simulink model "UAM_Flight_control"  (R2024b)
settings: Solver=FixedStepAuto  StartTime=0.0  StopTime=inf  RelTol=1e-3  EnableMultiTasking=on
undefined symbols (not defined in the file): CityMission, control, controlParams, ControlSampleTime, Cruise_a, DiscIntNeverNeededParam, Earth, FixedWingMission, flightState, FSState, FWControlParams, FWTrimSpeed, HoverMission, params, position, R_WAYPOINTTRANSITION, TransitionMission, uavParam, Vt, w_trim, WGS84, zGround
libraries: slpidlib x56, simulink x35, uavalgslib x8, robotcorelib x2, simulink_extras x2, mspfiltlib x1, aerolibtransform2 x1
(part 2 of 12)

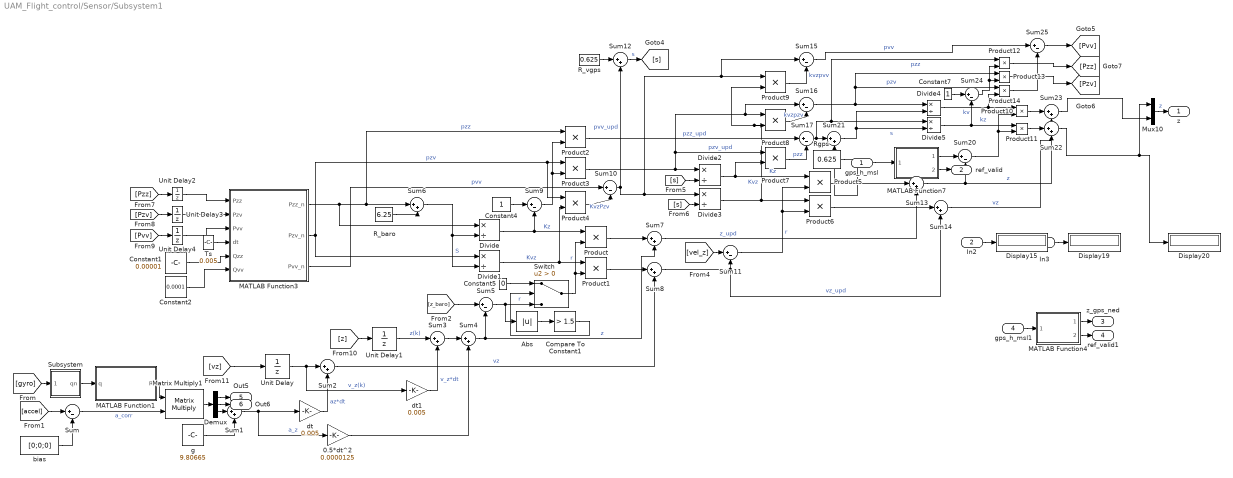
== system UAM_Flight_control/Sensor/Subsystem1 ==
  gps_h_msl : Inport
  In2 : Inport  Port=2
  In3 : Inport  Port=3
  gps_h_msl1 : Inport  Port=4
  0.5*dt^2 : Gain  Gain=0.0000125
  Abs : Abs  SaturateOnIntegerOverflow=off
  Compare To Constant1 : simulink/Logic and Bit Operations/Compare To Constant  relop=>  const=1.5  OutDataTypeStr=boolean
  Constant1 : Constant  Value=0.00001
  Constant2 : Constant  Value=0.0001
  Constant4 : Constant
  Constant5 : Constant  Value=0
  Constant7 : Constant
  Demux : Demux  Outputs=3
  Display15 : Display
  Display19 : Display
  Display20 : Display
  Divide{,1..5} (6 alike) : Product  Inputs=*/
  MATLAB Function1 : MATLAB Function  TreatAsAtomicUnit=on
  MATLAB Function3 : MATLAB Function  TreatAsAtomicUnit=on
  MATLAB Function4 : MATLAB Function  TreatAsAtomicUnit=on
  MATLAB Function7 : MATLAB Function  TreatAsAtomicUnit=on
  Matrix Multiply1 : Product  Multiplication=Matrix(*)
  Mux10 : Mux  Inputs=2
  Product{,1..14} (15 alike) : Product
  R_baro : Constant  Value=6.25
  R_vgps : Constant  Value=0.625
  Rgps : Constant  Value=0.625
  Subsystem : Subsystem
  Sum{,5,9..11,15..17,20,24..25} (11 alike) : Sum  Inputs=|+-
  Sum{1..4,6..8,12..14,21..23} (13 alike) : Sum  Inputs=|++
  Switch : Switch  Criteria=u2 > Threshold  SaturateOnIntegerOverflow=off  InputSameDT=off
  Ts : Constant  Value=0.005
  Unit Delay{,1..4} (5 alike) : UnitDelay  SampleTime=-1  HasFrameUpgradeWarning=on
  bias : Constant  Value=[0;0;0]
  dt : Gain  Gain=0.005
  dt1 : Gain  Gain=0.005
  g : Constant  Value=9.80665
  z : Outport
  ref_valid : Outport  Port=2
  z_gps_ned : Outport  Port=3
  ref_valid1 : Outport  Port=4
  Out5 : Outport  Port=5
  Out6 : Outport  Port=6
  wires:
  Sum1/1 -> dt/1, 0.5*dt^2/1  "a_z"
  Sum10/1 -> Sum12/2, Product9/1, Sum15/1, Divide3/1  "pvv_upd"
  In2/1 -> Display15/1
  Constant5/1 -> Switch/1
  Sum6/1 -> Divide1/2, Divide/2  "S"
  Unit Delay/1 -> dt1/1, Sum2/1  "v_z(k)"
  gps_h_msl1/1 -> MATLAB Function4/1(gps_h_msl)
  Divide2/1 -> Product7/2, Product5/1  "Kz"
  Product9/1 -> Sum15/2  "kvzpvv"
  Sum16/1 -> Product13/1, Product14/1, Divide4/1  "pzv"
  dt1/1 -> Sum3/2  "v_z*dt"
  [vz] -> Unit Delay/1
  [Pzv] -> Unit Delay3/1
  Divide4/1 -> Product14/2, Product10/1  "kv"
  Ts/1 -> MATLAB Function3/4(dt)
  bias/1 -> Sum/2
  Sum13/1 -> Sum22/2, Sum20/2  "z"
  MATLAB Function7/1(z_gps_ned) -> Sum20/1
  Matrix Multiply1/1 -> Demux/1
  [Pzz] -> Unit Delay2/1
  Compare To Constant1/1 -> Switch/2
  [z] -> Unit Delay1/1
  g/1 -> Sum1/2
  Sum20/1 -> Product11/2, Product10/2
  Product12/1 -> [Pzz]
  Abs/1 -> Compare To Constant1/1
  Unit Delay2/1 -> MATLAB Function3/1(Pzz)
  Divide3/1 -> Product9/2, Product8/2, Product6/1  "Kvz"
  Sum9/1 -> Product2/2, Product3/2
  Sum/1 -> Matrix Multiply1/2  "a_corr"
  Sum7/1 -> Sum13/2  "z_upd"
  Sum23/1 -> Mux10/2
  Product5/1 -> Sum13/1
  Sum4/1 -> Sum7/2, Sum5/2  "z"
  Sum22/1 -> Display20/1, Mux10/1
  Sum21/1 -> Divide5/2, Divide4/2  "s"
  Sum2/1 -> Sum8/2  "vz"
  R_baro/1 -> Sum6/2
  Sum17/1 -> Product12/1, Divide5/1, Sum21/1  "pzz"
  MATLAB Function3/3(Pvv_n) -> Sum10/1  "pvv"
  dt/1 -> Sum2/2  "az*dt"
  Divide1/1 -> Product1/1, Product4/2  "Kvz"
  Product13/1 -> [Pzv]
  Constant2/1 -> MATLAB Function3/6(Qvv)
  Sum5/1 -> Switch/3, Abs/1  "r"
  Sum25/1 -> [Pvv]
  Product/1 -> Sum7/1
  Sum11/1 -> Product6/2, Product5/2  "r"
  Product10/1 -> Sum23/1
  Sum3/1 -> Sum4/1
  MATLAB Function3/2(Pzv_n) -> Divide1/1, Product4/1, Product3/1  "pzv"
  Sum8/1 -> Sum14/2, Sum11/2  "vz_upd"
  [gyro] -> Subsystem/1(Inport)
  Subsystem/1(qn) -> MATLAB Function1/1(q)
  MATLAB Function7/2(ref_valid) -> ref_valid/1
  [accel] -> Sum/1
  MATLAB Function3/1(Pzz_n) -> Divide/1, Product2/1, Sum6/1  "pzz"
  Product8/1 -> Sum16/2  "kvzpzv"
  Sum15/1 -> Sum25/1  "pvv"
  Product7/1 -> Sum17/2  "pzz"
  Unit Delay4/1 -> MATLAB Function3/3(Pvv)
  Rgps/1 -> Sum21/2
  Divide5/1 -> Product11/1, Sum24/2  "kz"
  Product3/1 -> Sum16/1, Product8/1, Product7/1, Divide2/1  "pzv_upd"
  Switch/1 -> Product/2, Product1/2  "r"
  Product4/1 -> Sum10/2  "KvzPzv"
  Unit Delay3/1 -> MATLAB Function3/2(Pzv)
  Unit Delay1/1 -> Sum3/1  "z(k)"
  Divide/1 -> Sum9/2, Product/1  "Kz"
  [vel_z] -> Sum11/1
  [s] -> Divide2/2
  Product11/1 -> Sum22/1
  Demux/3 -> Sum1/1
  Constant1/1 -> MATLAB Function3/5(Qzz)
  Sum24/1 -> Product13/2, Product12/2
  Constant4/1 -> Sum9/1
  R_vgps/1 -> Sum12/1
  [s] -> Divide3/2
  Sum12/1 -> [s]  "s"
  Product1/1 -> Sum8/1
  Product14/1 -> Sum25/2
  Sum14/1 -> Sum23/2  "vz"
  [Pvv] -> Unit Delay4/1
  Product6/1 -> Sum14/1
  MATLAB Function1/1(R) -> Matrix Multiply1/1
  Product2/1 -> Sum17/1  "pzz_upd"
  0.5*dt^2/1 -> Sum4/2
  Constant7/1 -> Sum24/1
  [z_baro] -> Sum5/1
  gps_h_msl/1 -> MATLAB Function7/1(gps_h_msl)
  In3/1 -> Display19/1
  MATLAB Function4/1(z_gps_ned) -> z_gps_ned/1
  MATLAB Function4/2(ref_valid) -> ref_valid1/1
  Demux/2 -> Out6/1
  Mux10/1 -> z/1  "z"
  Demux/1 -> Out5/1

== system UAM_Flight_control/Sensor/Subsystem2 ==
  fcc : Inport
  In2 : Inport  Port=2
  Constant1 : Constant  Value=0
  Gain : Gain  Gain=pi/180
  Gain1 : Gain  Gain=pi/180
  Matrix Concatenate : Concatenate  NumInputs=3  Mode=Multidimensional array  ConcatenateDimension=2
  Product{,1..3} (4 alike) : Product
  Trigonometric Function : Trigonometry
  Trigonometric Function1 : Trigonometry  Operator=cos
  Trigonometric Function2 : Trigonometry  Operator=cos
  Trigonometric Function3 : Trigonometry
  Unary Minus{,1..5} (6 alike) : UnaryMinus
  Vector Concatenate : Concatenate  NumInputs=3
  Vector Concatenate1 : Concatenate  NumInputs=3
  Vector Concatenate2 : Concatenate  NumInputs=3
  Out1 : Outport
  wires:
  Product3/1 -> Unary Minus3/1
  Vector Concatenate/1 -> Matrix Concatenate/1
  Trigonometric Function1/1 -> Vector Concatenate1/2, Product3/2, Product/2, Product2/2
  Unary Minus4/1 -> Vector Concatenate2/3
  Vector Concatenate2/1 -> Matrix Concatenate/3
  Trigonometric Function3/1 -> Unary Minus5/1, Product1/2
  Trigonometric Function/1 -> Product1/1, Unary Minus4/1, Product/1
  Gain/1 -> Trigonometric Function2/1, Trigonometric Function/1
  Product/1 -> Unary Minus/1
  Vector Concatenate1/1 -> Matrix Concatenate/2
  Trigonometric Function2/1 -> Product2/1, Product3/1, Vector Concatenate/3
  fcc/1 -> Gain/1
  Gain1/1 -> Trigonometric Function1/1, Trigonometric Function3/1
  Constant1/1 -> Vector Concatenate1/3
  Unary Minus5/1 -> Vector Concatenate1/1
  In2/1 -> Gain1/1
  Unary Minus2/1 -> Vector Concatenate2/1
  Product2/1 -> Unary Minus2/1
  Product1/1 -> Unary Minus1/1
  Unary Minus/1 -> Vector Concatenate/1
  Unary Minus1/1 -> Vector Concatenate/2
  Unary Minus3/1 -> Vector Concatenate2/2
  Matrix Concatenate/1 -> Out1/1

== system UAM_Flight_control/Controller/Auto1/Blend Scheduler ==
  note: Forward Transition Tilt Mode Manager
  FlightMode : Inport
  States : Inport  Port=2
  MixerCommands : Inport  Port=3
  BTalpha : Subsystem  TreatAsAtomicUnit=on
  Bus Creator : BusCreator  Inputs=5
  Bus Selector1 : BusSelector  OutputSignals=w_phi,w_theta,w_psi,w_z
  Constant : Constant  Value=flightState.Transition
  Constant2 : Constant  Value=0.25*uavParam.geom.mass*9.81
  Constant3 : Constant  Value=FWTrimSpeed
  Constant4 : Constant  Value=FWTrimSpeed
  Constant5 : Constant
  Constant6 : Constant  Value=78.54
  Constant7 : Constant
  Demux : Demux
  FTalpha : Subsystem
  Gain3 : Gain  Gain=0
  Mux : Mux
  Product1 : Product
  Product2 : Product
  Product3 : Product
  Relational Operator : RelationalOperator  Operator===  OutDataTypeStr=boolean  RndMeth=Simplest  InputSameDT=off
  Subtract : Sum  Inputs=+-
  Subtract1 : Sum  Inputs=+-
  Sum1 : Sum  Inputs=|++
  Sum3 : Sum  Inputs=|+-
  Switch : Switch  Criteria=u2 > Threshold  SaturateOnIntegerOverflow=off  InputSameDT=off
  Switch1 : Switch  Criteria=u2 > Threshold  SaturateOnIntegerOverflow=off  InputSameDT=off
  MotorCommands : Outport
  alpha : Outport  Port=2
  FlightState : Outport  Port=3
  wires:
  FlightMode/1 -> Relational Operator/1, FlightState/1
  Relational Operator/1 -> [trigger]
  Bus Selector1/4 -> Sum1/1  "<w_z>"
  Constant2/1 -> Sum1/2
  [liftblending] -> Product2/2
  Mux/1 -> Product2/1
  MixerCommands/1 -> Bus Selector1/1
  Bus Selector1/1 -> Mux/1  "<w_phi>"
  Bus Selector1/2 -> Mux/2  "<w_theta>"
  Bus Selector1/3 -> Mux/3  "<w_psi>"
  Sum1/1 -> Mux/4  "w_z"
  Product2/1 -> Demux/1
  Demux/1 -> Bus Creator/1  "w_phi"
  Demux/2 -> Bus Creator/2  "w_theta"
  Demux/3 -> Bus Creator/3  "w_psi"
  Demux/4 -> Bus Creator/4  "w_z"
  Bus Creator/1 -> MotorCommands/1
  Constant6/1 -> Product1/1
  States/1 -> FTalpha/1(States), BTalpha/1(States)
  Switch/1 -> [liftblending], Subtract1/2
  FTalpha/1(alpha) -> Switch/1
  BTalpha/1(alpha) -> Switch/3
  [trigger] -> Switch/2
  Product1/1 -> Sum3/2
  Sum3/1 -> Switch1/1  "cruise"
  [trigger] -> Switch1/2
  Switch1/1 -> Bus Creator/5  "cruise"
  Constant3/1 -> Gain3/1
  Gain3/1 -> Product3/1
  Constant5/1 -> Subtract/1
  [liftblending] -> Subtract/2
  Subtract/1 -> Product3/2
  Product3/1 -> Switch1/3
  Constant7/1 -> Subtract1/1
  Subtract1/1 -> alpha/1
  Constant/1 -> Relational Operator/2
  [liftblending] -> Product1/2
  Constant4/1 -> Sum3/1

== system UAM_Flight_control/Controller/Auto1/Fixed Wing Controller ==
  States : Inport
  Control Mode : Inport  Port=2
  AAC SP : Inport  Port=3  OutDataTypeStr=Bus: AAC
  FixedWingSP : Inport  Port=4  OutDataTypeStr=Bus: FixedWingCommandBus
  AERT : Inport  Port=5
  In1 : Inport  Port=6
  Actuator Armed : EnablePort
  Subsystem : Subsystem
  Actuator : Outport
  wires:
  States/1 -> Subsystem/1(States)
  Control Mode/1 -> Subsystem/2(Control Mode)
  AAC SP/1 -> Subsystem/3(AAC SP)
  Subsystem/1(Actuator) -> Actuator/1
  AERT/1 -> Subsystem/5(AERT)
  FixedWingSP/1 -> Subsystem/4(FixedWingSP)
  In1/1 -> Subsystem/6(Intransition)

== system UAM_Flight_control/Controller/Auto1/Manual Control ==
  Bus Creator : BusCreator  Inputs=4
  Constant{,1..3} (4 alike) : Constant  Value=0  SampleTime=-1
  AERT : Outport
  wires:
  Constant/1 -> Bus Creator/1  "aileron"
  Constant1/1 -> Bus Creator/2  "throttle"
  Constant2/1 -> Bus Creator/3  "elevator"
  Constant3/1 -> Bus Creator/4  "rudder"
  Bus Creator/1 -> AERT/1

== system UAM_Flight_control/Controller/Auto1/Multicopter Controller ==
  note: Prefilter
  Hover Commands : Inport  OutDataTypeStr=Bus: HoverSPBus
  States : Inport  Port=2
  InTransition : Inport  Port=3
  CtrlMode : Inport  Port=4
  FlightMode : Inport  Port=5
  " Armed" : EnablePort
  Attitude & Altitude controller : Subsystem
  Demux1 : Demux
  Horizontal Position Control : Subsystem  TreatAsAtomicUnit=on
  Merge : Merge
  Merge1 : Merge
  Mux : Mux  Inputs=3
  NOT1 : Logic  Operator=NOT  IconShape=distinctive  AllPortsSameDT=off  OutDataTypeStr=boolean
  Organize Inputs : Subsystem
  transition controller : Subsystem
  MixerCommands : Outport
  wires:
  Organize Inputs/1(MixerCommands) -> MixerCommands/1
  Demux1/1 -> [XRef]
  [State] -> Horizontal Position Control/3(States)
  Demux1/3 -> [ZRef]
  NOT1/1 -> Horizontal Position Control/Enable
  [XRef] -> Horizontal Position Control/1(XRef)
  [YRef] -> Horizontal Position Control/2(YRef)
  InTransition/1 -> [Transition]
  States/1 -> [State]
  Hover Commands/1 -> Demux1/1
  Demux1/4 -> [YawRef]
  Mux/1 -> Attitude & Altitude controller/1(Ref Attitude)
  [State] -> Attitude & Altitude controller/2(States)
  [ZRef] -> Attitude & Altitude controller/3(Z ref)
  [Transition] -> Attitude & Altitude controller/4(InTransition)
  Attitude & Altitude controller/1(Roll torque cmd) -> Organize Inputs/2(commanded phi torque)
  Attitude & Altitude controller/2(Pitch torque Cmd) -> Organize Inputs/3(commanded theta torque)
  Attitude & Altitude controller/4(commanded thrust) -> Organize Inputs/5(commanded thrust)
  FlightMode/1 -> Attitude & Altitude controller/6(FlightMode)
  Attitude & Altitude controller/3(Yaw torque Cmd) -> Organize Inputs/4(commanded psi torque)
  [Transition] -> NOT1/1, transition controller/Enable
  [YawRef] -> Mux/3
  Demux1/2 -> [YRef]
  Merge/1 -> Mux/1
  Merge1/1 -> Mux/2
  transition controller/1(Rollcmd) -> Merge/2
  transition controller/2(Pitchcmd) -> Merge1/2
  Horizontal Position Control/1(Roll Cmd) -> Merge/1
  Horizontal Position Control/2(Pitch Cmd) -> Merge1/1
  CtrlMode/1 -> Attitude & Altitude controller/5(CtrlMode)

== system UAM_Flight_control/Controller/Auto1/Scheduler ==
  MotorCommands : Inport
  FlightState : Inport  Port=2  OutDataTypeStr=Enum: flightState
  CtrlMode : Inport  Port=3
  FixedWingActuators : Inport  Port=4
  " Armed" : EnablePort
  FixedWingScheduler : Subsystem
  Subsystem : Subsystem
  MotorActuatorCommands : Outport  OutputWhenDisabled=reset  InitialOutput=0
  CtrlSurfaceCommands : Outport  Port=2  OutDataTypeStr=Bus: FixedWingCtrlBus  OutputWhenDisabled=reset  InitialOutput=0  VectorParamsAs1DForOutWhenUnconnected=off
  wires:
  FixedWingScheduler/1(ActuatorControls) -> CtrlSurfaceCommands/1, Subsystem/2(FixedWingActuators)
  FlightState/1 -> Subsystem/1(FlightState), FixedWingScheduler/1(FlightState)
  Subsystem/1(ActuatorControls) -> MotorActuatorCommands/1
  MotorCommands/1 -> Subsystem/4(MotorCommands)
  FixedWingActuators/1 -> FixedWingScheduler/2(FixedWingActuators)
  CtrlMode/1 -> Subsystem/3(CtrlMode)

== system UAM_Flight_control/Controller/Emergency/Blend Scheduler ==
  FlightMode : Inport
  States : Inport  Port=2
  Constant : Constant  Value=flightState.Transition
  Constant1 : Constant  Value=flightState.BackTransition
  Discrete-Time Integrator : DiscreteIntegrator  gainval=0.01  SampleTime=-1  ICPrevOutput=DiscIntNeverNeededParam  ICPrevScaledInput=DiscIntNeverNeededParam
  Gain : Gain
  Gain1 : Gain  Gain=-1
  Relational Operator : RelationalOperator  Operator===  OutDataTypeStr=boolean  RndMeth=Simplest  InputSameDT=off
  Relational Operator1 : RelationalOperator  Operator===  OutDataTypeStr=boolean  RndMeth=Simplest  InputSameDT=off
  Saturation : Saturate  UpperLimit=1  LowerLimit=0  OutDataTypeStr=double
  Sum : Sum  Inputs=|++
  Terminator : Terminator
  alpha : Outport
  FlightState : Outport  Port=2
  wires:
  FlightMode/1 -> Relational Operator1/1, Relational Operator/1, FlightState/1
  Gain/1 -> Sum/1
  Gain1/1 -> Sum/2
  Sum/1 -> Discrete-Time Integrator/1
  Discrete-Time Integrator/1 -> Saturation/1
  Saturation/1 -> alpha/1  "a"
  States/1 -> Terminator/1
  Constant/1 -> Relational Operator/2
  Relational Operator/1 -> Gain/1
  Constant1/1 -> Relational Operator1/2
  Relational Operator1/1 -> Gain1/1

== system UAM_Flight_control/Controller/Emergency/FixedWing Controller ==
  States : Inport
  Control Mode : Inport  Port=2
  RC : Inport  Port=3
  Actuator Armed : EnablePort
  Subsystem : Subsystem
  Actuator : Outport
  wires:
  States/1 -> Subsystem/1(States)
  Control Mode/1 -> Subsystem/2(Control Mode)
  Subsystem/1(Actuator) -> Actuator/1
  RC/1 -> Subsystem/3(RC)

== system UAM_Flight_control/Controller/Emergency/Scheduler ==
  MotorCommands : Inport
  BlendingSchedule : Inport  Port=2
  FlightState : Inport  Port=3  OutDataTypeStr=Enum: flightState
  TransitionDone : Inport  Port=4
  BackTransitionDone : Inport  Port=5
  FixedWingActuators : Inport  Port=6  OutDataTypeStr=Bus: FixedWingCtrlBus
  Actuator Armed : EnablePort
  FixedWingScheduler : Subsystem
  Subsystem : Subsystem
  MotorActuatorCommands : Outport  OutputWhenDisabled=reset  InitialOutput=0
  CtrlSurfaceCommands : Outport  Port=2  OutDataTypeStr=Bus: FixedWingCtrlBus  OutputWhenDisabled=reset  InitialOutput=0  VectorParamsAs1DForOutWhenUnconnected=off
  wires:
  FixedWingScheduler/1(ActuatorControls) -> CtrlSurfaceCommands/1, Subsystem/2(FixedWingActuators)
  FlightState/1 -> Subsystem/1(FlightState), FixedWingScheduler/1(FlightState)
  BlendingSchedule/1 -> Subsystem/4(BlendingSchedule)
  Subsystem/1(ActuatorControls) -> MotorActuatorCommands/1
  MotorCommands/1 -> Subsystem/3(MotorCommands)
  FixedWingActuators/1 -> FixedWingScheduler/2(FixedWingActuators)
  TransitionDone/1 -> Subsystem/5(TransitionDone), FixedWingScheduler/3(TransitionDone)
  BackTransitionDone/1 -> Subsystem/6(BackTransitionDone)

== system UAM_Flight_control/Controller/Emergency/multicopter Controller ==
  RC : Inport
  States : Inport  Port=2
  Actuator Armed : EnablePort
  Attitude & Altitude controller : Subsystem
  Demux : Demux  Outputs=10
  Mux1 : Mux  Inputs=3
  Organize Inputs : Subsystem
  Terminator{,1..6} (7 alike) : Terminator
  MixerCommands : Outport
  wires:
  Demux/6 -> Terminator2/1
  Organize Inputs/1(MixerCommands) -> MixerCommands/1
  Demux/2 -> Organize Inputs/1(forward command), Mux1/2
  Demux/5 -> Terminator1/1
  Attitude & Altitude controller/3(Yaw torque Cmd) -> Organize Inputs/4(commanded psi torque)
  States/1 -> Attitude & Altitude controller/2(States)
  Demux/4 -> Mux1/3
  Attitude & Altitude controller/1(Roll torque cmd) -> Organize Inputs/2(commanded phi torque)
  Attitude & Altitude controller/2(Pitch torque Cmd) -> Organize Inputs/3(commanded theta torque)
  Attitude & Altitude controller/4(commanded thrust) -> Organize Inputs/5(commanded thrust)
  Demux/1 -> Mux1/1
  Mux1/1 -> Attitude & Altitude controller/1(Ref Attitude)
  Demux/3 -> Terminator/1
  RC/1 -> Demux/1
  Demux/7 -> Terminator3/1
  Demux/8 -> Terminator4/1
  Demux/9 -> Terminator5/1
  Demux/10 -> Terminator6/1

== system UAM_Flight_control/Controller/Manual/Blend Scheduler ==
  FlightMode : Inport
  States : Inport  Port=2
  Constant : Constant  Value=flightState.Transition
  Constant1 : Constant  Value=flightState.BackTransition
  Discrete-Time Integrator : DiscreteIntegrator  gainval=0.01  SampleTime=-1  ICPrevOutput=DiscIntNeverNeededParam  ICPrevScaledInput=DiscIntNeverNeededParam
  Gain : Gain
  Gain1 : Gain  Gain=-1
  Relational Operator : RelationalOperator  Operator===  OutDataTypeStr=boolean  RndMeth=Simplest  InputSameDT=off
  Relational Operator1 : RelationalOperator  Operator===  OutDataTypeStr=boolean  RndMeth=Simplest  InputSameDT=off
  Saturation : Saturate  UpperLimit=1  LowerLimit=0  OutDataTypeStr=double
  Sum : Sum  Inputs=|++
  Terminator : Terminator
  alpha : Outport
  FlightState : Outport  Port=2
  wires:
  FlightMode/1 -> Relational Operator1/1, Relational Operator/1, FlightState/1
  Gain/1 -> Sum/1
  Gain1/1 -> Sum/2
  Sum/1 -> Discrete-Time Integrator/1
  Discrete-Time Integrator/1 -> Saturation/1
  Saturation/1 -> alpha/1  "a"
  States/1 -> Terminator/1
  Constant/1 -> Relational Operator/2
  Relational Operator/1 -> Gain/1
  Constant1/1 -> Relational Operator1/2
  Relational Operator1/1 -> Gain1/1

== system UAM_Flight_control/Controller/Manual/FixedWing Controller ==
  States : Inport
  Control Mode : Inport  Port=2
  RC : Inport  Port=3
  Actuator Armed : EnablePort
  Subsystem : Subsystem
  Actuator : Outport
  wires:
  States/1 -> Subsystem/1(States)
  Control Mode/1 -> Subsystem/2(Control Mode)
  Subsystem/1(Actuator) -> Actuator/1
  RC/1 -> Subsystem/3(RC)

== system UAM_Flight_control/Controller/Manual/Scheduler ==
  MotorCommands : Inport
  BlendingSchedule : Inport  Port=2
  FlightState : Inport  Port=3  OutDataTypeStr=Enum: flightState
  TransitionDone : Inport  Port=4
  BackTransitionDone : Inport  Port=5
  FixedWingActuators : Inport  Port=6  OutDataTypeStr=Bus: FixedWingCtrlBus
  Actuator Armed : EnablePort
  FixedWingScheduler : Subsystem
  Subsystem : Subsystem
  MotorActuatorCommands : Outport  OutputWhenDisabled=reset  InitialOutput=0
  CtrlSurfaceCommands : Outport  Port=2  OutDataTypeStr=Bus: FixedWingCtrlBus  OutputWhenDisabled=reset  InitialOutput=0  VectorParamsAs1DForOutWhenUnconnected=off
  wires:
  FixedWingScheduler/1(ActuatorControls) -> CtrlSurfaceCommands/1, Subsystem/2(FixedWingActuators)
  FlightState/1 -> Subsystem/1(FlightState), FixedWingScheduler/1(FlightState)
  BlendingSchedule/1 -> Subsystem/4(BlendingSchedule)
  Subsystem/1(ActuatorControls) -> MotorActuatorCommands/1
  MotorCommands/1 -> Subsystem/3(MotorCommands)
  FixedWingActuators/1 -> FixedWingScheduler/2(FixedWingActuators)
  TransitionDone/1 -> Subsystem/5(TransitionDone), FixedWingScheduler/3(TransitionDone)
  BackTransitionDone/1 -> Subsystem/6(BackTransitionDone)

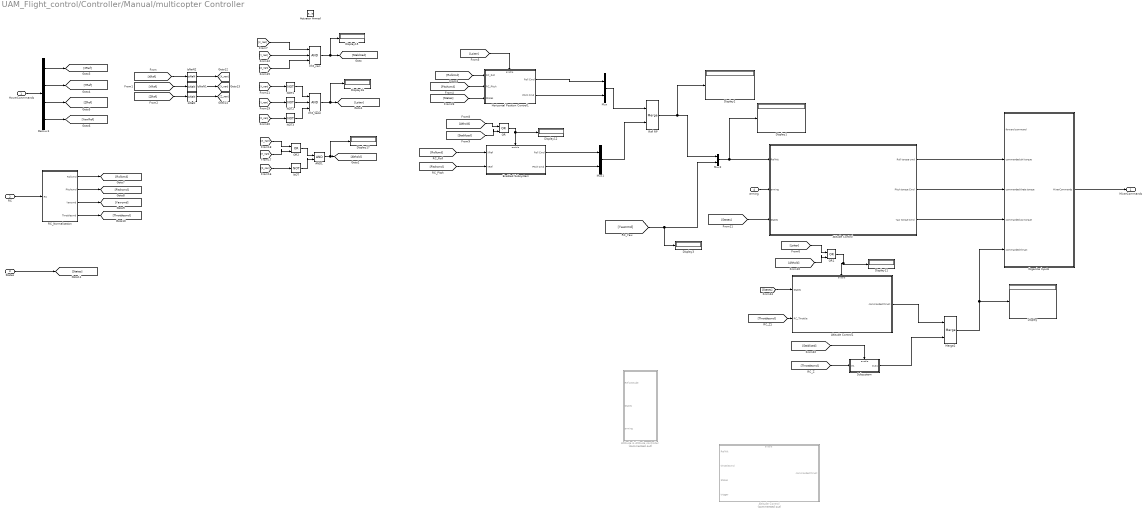
== system UAM_Flight_control/Controller/Manual/multicopter Controller ==
  HoverConmmands : Inport
  RC : Inport  Port=2
  States : Inport  Port=3
  arming : Inport  Port=4
  Actuator Armed : EnablePort
  AND1 : Logic  IconShape=distinctive  AllPortsSameDT=off  OutDataTypeStr=boolean
  Altitude Control : Subsystem  Commented=on
  Altitude Control1 : Subsystem
  Atitude Control : Subsystem
  Attitude & Altitude controller : Subsystem  Commented=on
  Demux1 : Demux
  Display{,1..3,11..12,15..17} (9 alike) : Display
  Enabled Subsystem : Subsystem  TreatAsAtomicUnit=on
  Horizontal Position Control1 : Subsystem  TreatAsAtomicUnit=on
  IsNaN : RelationalOperator  Operator=isNaN  OutDataTypeStr=boolean  RndMeth=Simplest  InputSameDT=off
  IsNaN1 : RelationalOperator  Operator=isNaN  OutDataTypeStr=boolean  RndMeth=Simplest  InputSameDT=off
  IsNaN2 : RelationalOperator  Operator=isNaN  OutDataTypeStr=boolean  RndMeth=Simplest  InputSameDT=off
  Merge2 : Merge
  Mux : Mux  Inputs=2
  Mux1 : Mux  Inputs=2
  Mux2 : Mux  Inputs=2
  NOT{,1..3} (4 alike) : Logic  Operator=NOT  IconShape=distinctive  AllPortsSameDT=off  OutDataTypeStr=boolean
  OR : Logic  Operator=OR  IconShape=distinctive  AllPortsSameDT=off  OutDataTypeStr=boolean
  OR1 : Logic  Operator=OR  IconShape=distinctive  AllPortsSameDT=off  OutDataTypeStr=boolean
  OR2 : Logic  Operator=OR  IconShape=distinctive  AllPortsSameDT=off  OutDataTypeStr=boolean
  Organize Inputs : Subsystem
  RC_Normalization : Subsystem
  Ref RP : Merge
  Subsystem : Subsystem
  XYZ_Valid : Logic  Inputs=3  IconShape=distinctive  AllPortsSameDT=off  OutDataTypeStr=boolean
  XYZ_nan : Logic  Inputs=3  IconShape=distinctive  AllPortsSameDT=off  OutDataTypeStr=boolean
  MixerCommands : Outport
  wires:
  Organize Inputs/1(MixerCommands) -> MixerCommands/1
  HoverConmmands/1 -> Demux1/1
  Demux1/1 -> [XRef]
  Demux1/2 -> [YRef]
  Demux1/3 -> [ZRef]
  Demux1/4 -> [YawRef]
  [XRef] -> IsNaN2/1
  [YRef] -> IsNaN1/1
  [ZRef] -> IsNaN/1
  RC/1 -> RC_Normalization/1(RC)
  RC_Normalization/1(Rollcmd) -> [Rollcmd]
  RC_Normalization/2(Pitchcmd) -> [Pitchcmd]
  RC_Normalization/3(Yawcmd) -> [Yawcmd]
  RC_Normalization/4(Throttlecmd) -> [Throttlecmd]
  [Rollcmd] -> Enabled Subsystem/1(XRef)
  [Pitchcmd] -> Enabled Subsystem/2(YRef)
  Enabled Subsystem/1(Roll Cmd) -> Mux1/1
  Enabled Subsystem/2(Pitch Cmd) -> Mux1/2
  Mux1/1 -> Ref RP/2
  OR/1 -> Enabled Subsystem/Enable, Display12/1
  [Althold] -> OR/1
  [Stablized] -> OR/2
  Ref RP/1 -> Display2/1, Mux2/1
  [Yawcmd] -> Display3/1, Mux2/2
  Mux2/1 -> Atitude Control/1(Ref Att), Display1/1
  arming/1 -> Atitude Control/2(arming)
  States/1 -> [States]
  Atitude Control/1(Roll torque cmd) -> Organize Inputs/2(commanded phi torque)
  Atitude Control/2(Pitch torque Cmd) -> Organize Inputs/3(commanded theta torque)
  Atitude Control/3(Yaw torque Cmd) -> Organize Inputs/4(commanded psi torque)
  [States] -> Atitude Control/3(States)
  Merge2/1 -> Organize Inputs/5(commanded thrust), Display/1
  [Loiter] -> OR1/1
  OR1/1 -> Altitude Control1/Enable, Display11/1
  [Althold] -> OR1/2
  AND1/1 -> Display17/1, [Althold]
  IsNaN2/1 -> [X_nan]
  IsNaN1/1 -> [Y_nan]
  IsNaN/1 -> [Z_nan]
  [X_nan] -> XYZ_nan/1
  [Y_nan] -> XYZ_nan/2
  [Z_nan] -> XYZ_nan/3
  [Z_nan] -> NOT/1
  NOT/1 -> AND1/2
  OR2/1 -> AND1/1
  [X_nan] -> OR2/1
  [Y_nan] -> OR2/2
  [X_nan] -> NOT1/1
  NOT1/1 -> XYZ_Valid/1
  NOT2/1 -> XYZ_Valid/2
  [Y_nan] -> NOT2/1
  [Z_nan] -> NOT3/1
  NOT3/1 -> XYZ_Valid/3
  XYZ_Valid/1 -> Display16/1, [Loiter]
  [Throttlecmd] -> Subsystem/1(In1)
  Subsystem/1(Out1) -> Merge2/2
  [Stablized] -> Subsystem/Enable
  Mux/1 -> Ref RP/1
  XYZ_nan/1 -> Display15/1, [Stablized]
  [States] -> Altitude Control1/1(States)
  [Throttlecmd] -> Altitude Control1/2(RC_Throttle)
  Altitude Control1/1(commanded thrust) -> Merge2/1
  Horizontal Position Control1/2(Pitch Cmd) -> Mux/2
  Horizontal Position Control1/1(Roll Cmd) -> Mux/1
  [States] -> Horizontal Position Control1/3(States)
  [Rollcmd] -> Horizontal Position Control1/1(RC_Roll)
  [Pitchcmd] -> Horizontal Position Control1/2(RC_Pitch)
  [Loiter] -> Horizontal Position Control1/Enable

== system UAM_Flight_control/Flightmode/Auto/Guidance Mode Selector/GuidanceLogic.BackTransition ==
  States : Inport  OutDataTypeStr=Bus: GuidanceStates
  Action Port : ActionPort
      settings: CopyFcn=Stateflow.SLINSF.SimulinkMan.removeBlockPreDeleteFcn  PreDeleteFcn=Stateflow.SLINSF.SimulinkMan.unsafePredeleteFcn
  Bus Creator1 : BusCreator  Inputs=3  OutDataTypeStr=Bus: innerLoopCmdsBus  NonVirtualBus=on
  Bus Selector : BusSelector  OutputSignals=Xe
  Constant : Constant  Value=0
  Constant1 : Constant  Value=0
  Constant2 : Constant  Value=0
  Data Type Conversion : DataTypeConversion  OutDataTypeStr=uint8  SaturateOnIntegerOverflow=off  RndMeth=Floor
  Gain : Gain
  Status : Outport
  InnerLoopCmds : Outport  Port=2  OutDataTypeStr=Bus: innerLoopCmdsBus
  wires:
  States/1 -> Bus Selector/1
  Bus Selector/1 -> Gain/1  "<Xe>"
  Bus Creator1/1 -> InnerLoopCmds/1
  Constant1/1 -> Bus Creator1/2  "HeadingCmd"
  Constant2/1 -> Bus Creator1/3  "YawCmd"
  Data Type Conversion/1 -> Status/1
  Gain/1 -> Bus Creator1/1  "LAP"
  Constant/1 -> Data Type Conversion/1

== system UAM_Flight_control/Flightmode/Auto/Guidance Mode Selector/GuidanceLogic.FIXED_WING_ORBIT.ORBIT ==
  ToWP : Inport  OutDataTypeStr=Bus: UAVPathManagerBus
  States : Inport  Port=2
  Action Port : ActionPort
      settings: CopyFcn=Stateflow.SLINSF.SimulinkMan.removeBlockPreDeleteFcn  PreDeleteFcn=Stateflow.SLINSF.SimulinkMan.unsafePredeleteFcn
  Abs1 : Abs  SaturateOnIntegerOverflow=off
  Bus Creator : BusCreator  Inputs=5  OutDataTypeStr=Bus: AAC  NonVirtualBus=on
      settings: InheritFromInputs=off
  Bus Selector : BusSelector  OutputSignals=position,params
  Bus Selector1 : BusSelector  OutputSignals=Xe,course  OutputAsBus=on
  Bus to Vector : BusToVector
  Constant : Constant  Value=control.cruiseSpeed
  Constant1 : Constant  Value=0
  Data Type Conversion : DataTypeConversion  OutDataTypeStr=uint8  SaturateOnIntegerOverflow=off  RndMeth=Floor
  Lookahead Distance : Constant  Value=control.L1  OutDataTypeStr=double
  Relational Operator : RelationalOperator  Operator=>  OutDataTypeStr=boolean  RndMeth=Simplest  InputSameDT=off
  Selector : Selector  InputPortWidth=3  IndexOptions=Index vector (dialog)  Indices=3  OutputSizes=1
  Selector1 : Selector  InputPortWidth=4  IndexOptions=Index vector (dialog)  Indices=2  OutputSizes=1
  Selector2 : Selector  InputPortWidth=4  IndexOptions=Index vector (dialog)  Indices=1  OutputSizes=1
  Selector3 : Selector  InputPortWidth=4  IndexOptions=Index vector (dialog)  Indices=3  OutputSizes=1
  Terminator{,1..3} (4 alike) : Terminator
  UAV Orbit Follower : uavalgslib/Orbit Follower  UAVType=fixed-wing  MinOrbitRadius=control.turningRadius  MinLookaheadDistance=control.L1  ExternalReset=none  ShowCrossTrackErrorOutput=off  ShowNumTurnsOutput=on  SimulateUsing=Code generation
  Unary Minus : UnaryMinus
  Status : Outport
  aacSP : Outport  Port=2
  wires:
  Bus to Vector/1 -> UAV Orbit Follower/1
  Selector2/1 -> UAV Orbit Follower/3
  Bus Selector/1 -> UAV Orbit Follower/2, Selector/1  "<position>"
  ToWP/1 -> Bus Selector/1
  Bus Selector/2 -> Selector1/1, Selector3/1, Selector2/1  "<params>"
  Selector3/1 -> Relational Operator/2
  Relational Operator/1 -> Data Type Conversion/1
  UAV Orbit Follower/4 -> Terminator/1
  UAV Orbit Follower/5 -> Terminator1/1
  Bus Selector1/1 -> Bus to Vector/1
  States/1 -> Bus Selector1/1
  UAV Orbit Follower/1 -> Terminator2/1  "LAP"
  Lookahead Distance/1 -> UAV Orbit Follower/5, Bus Creator/4  "L1"
  Bus Creator/1 -> aacSP/1
  UAV Orbit Follower/2 -> Bus Creator/3  "course"
  Constant/1 -> Bus Creator/1  "airspeed"
  Unary Minus/1 -> Bus Creator/2  "altitude"
  UAV Orbit Follower/3 -> Terminator3/1  "YawCmd"
  Selector/1 -> Unary Minus/1
  UAV Orbit Follower/6 -> Abs1/1
  Abs1/1 -> Relational Operator/1
  Selector1/1 -> UAV Orbit Follower/4
  Constant1/1 -> Bus Creator/5  "climbrate"
  Data Type Conversion/1 -> Status/1

== system UAM_Flight_control/Flightmode/Auto/Guidance Mode Selector/GuidanceLogic.FIXED_WING_WAYPOINT.WAYPOINT ==
  note: This subsystem selects a lookahead point on the path and provides a desired course. Desired course is later converted to desired lateral acceleration (and roll setpoint)
  States : Inport  OutDataTypeStr=Bus: GuidanceStates
  ToWP : Inport  Port=2  OutDataTypeStr=Bus: UAVPathManagerBus
  FromWP : Inport  Port=3  OutDataTypeStr=Bus: UAVPathManagerBus
  Action Port : ActionPort
      settings: CopyFcn=Stateflow.SLINSF.SimulinkMan.removeBlockPreDeleteFcn  PreDeleteFcn=Stateflow.SLINSF.SimulinkMan.unsafePredeleteFcn
  Bus Creator : BusCreator  Inputs=5  OutDataTypeStr=Bus: AAC  NonVirtualBus=on
      settings: InheritFromInputs=off
  Bus Selector : BusSelector  OutputSignals=Xe,course  OutputAsBus=on
  Bus Selector1 : BusSelector  OutputSignals=position
  Bus Selector2 : BusSelector  OutputSignals=position
  Bus to Vector : BusToVector
  Constant : Constant  Value=control.cruiseSpeed
  Constant1 : Constant  Value=0
  Data Type Conversion : DataTypeConversion  SaturateOnIntegerOverflow=off  RndMeth=Floor
  Display{,2..4} (4 alike) : Display
  Lookahead Distance : Constant  Value=control.L1*15  OutDataTypeStr=double
  MATLAB Function : MATLAB Function  TreatAsAtomicUnit=on
  MATLAB Function1 : MATLAB Function  Commented=on  TreatAsAtomicUnit=on
  MATLAB Function2 : MATLAB Function  Commented=on  TreatAsAtomicUnit=on
  Scope : Scope
  Terminator : Terminator
  Terminator1 : Terminator
  Terminator2 : Terminator
  Waypoint Follower : uavalgslib/Waypoint Follower  UAVType=fixed-wing  StartFrom=first  TransitionRadiusSource=internal  TransitionRadius=FWControl.transitionRadius  MinLookaheadDistance=control.L1  HoverAtLastWaypoint=off  YawInput=off  ShowCrossTrackErrorOutput=off  ShowStatusOutput=on  SimulateUsing=Code generation
  Status : Outport
  aacSP : Outport  Port=2
  wires:
  Lookahead Distance/1 -> Waypoint Follower/3, Bus Creator/4  "L1"
  Waypoint Follower/1 -> Display4/1, Terminator/1  "LAP"
  Waypoint Follower/3 -> Terminator1/1  "YawCmd"
  Waypoint Follower/4 -> Terminator2/1
  Constant/1 -> Bus Creator/1  "airspeed"
  States/1 -> Bus Selector/1
  Bus Selector/1 -> Bus to Vector/1
  Waypoint Follower/5 -> Scope/1, Data Type Conversion/1
  Data Type Conversion/1 -> Status/1
  Bus Creator/1 -> aacSP/1
  ToWP/1 -> Bus Selector1/1
  FromWP/1 -> Bus Selector2/1
  Bus Selector1/1 -> MATLAB Function/1(toWP)  "<position>"
  Bus Selector2/1 -> MATLAB Function/2(fromWP)  "<position>"
  MATLAB Function/2(alt) -> Bus Creator/2
  Waypoint Follower/2 -> Display/1, Bus Creator/3  "course"
  Constant1/1 -> Bus Creator/5  "climbrate"
  Bus to Vector/1 -> Display3/1, Waypoint Follower/1
  MATLAB Function/1(wps) -> Display2/1, Waypoint Follower/2

== system UAM_Flight_control/Flightmode/Auto/Guidance Mode Selector/GuidanceLogic.ForwardTransition ==
  ToWP : Inport  OutDataTypeStr=Bus: UAVPathManagerBus
  FromWP : Inport  Port=2  OutDataTypeStr=Bus: UAVPathManagerBus
  Action Port : ActionPort
      settings: CopyFcn=Stateflow.SLINSF.SimulinkMan.removeBlockPreDeleteFcn  PreDeleteFcn=Stateflow.SLINSF.SimulinkMan.unsafePredeleteFcn
  Bus Creator : BusCreator  Inputs=5  OutDataTypeStr=Bus: AAC  NonVirtualBus=on
      settings: InheritFromInputs=off
  Bus Creator1 : BusCreator  Inputs=3  OutDataTypeStr=Bus: innerLoopCmdsBus  NonVirtualBus=on
  Bus Selector1 : BusSelector  OutputSignals=position
  Bus Selector2 : BusSelector  OutputSignals=position
  Constant : Constant  Value=0
  Constant1 : Constant  Value=0
  Constant2 : Constant  Value=0
  Constant3 : Constant  Value=[0 0 0]
  Data Type Conversion : DataTypeConversion  OutDataTypeStr=uint8  SaturateOnIntegerOverflow=off  RndMeth=Floor
  MATLAB Function : MATLAB Function  TreatAsAtomicUnit=on
  Switch : Switch  Criteria=u2 > Threshold  SaturateOnIntegerOverflow=off  InputSameDT=off
  Terminator : Terminator
  Status : Outport
  InnerLoopCmds : Outport  Port=2  OutDataTypeStr=Bus: innerLoopCmdsBus
  aacSP : Outport  Port=3
  wires:
  Bus Creator1/1 -> InnerLoopCmds/1
  Constant1/1 -> Bus Creator1/2  "HeadingCmd"
  Constant2/1 -> Bus Creator1/3  "YawCmd"
  Data Type Conversion/1 -> Status/1
  Constant/1 -> Data Type Conversion/1
  Constant3/1 -> Bus Creator1/1  "LAP"
  FromWP/1 -> Bus Selector2/1
  Bus Selector1/1 -> MATLAB Function/1(toWP)  "<position>"
  Bus Selector2/1 -> MATLAB Function/2(fromWP)  "<position>"
  ToWP/1 -> Bus Selector1/1
  Bus Creator/1 -> aacSP/1
  MATLAB Function/1(wps) -> Terminator/1
  MATLAB Function/2(alt) -> Bus Creator/2  "alt"

== system UAM_Flight_control/Flightmode/Auto/Guidance Mode Selector/GuidanceLogic.Land.AbortLoiter ==
  ToWP : Inport  OutDataTypeStr=Bus: UAVPathManagerBus
  Ground : Inport  Port=2
  Pose : Inport  Port=3
  FromWP : Inport  Port=4  OutDataTypeStr=Bus: UAVPathManagerBus
  Action Port : ActionPort
      settings: CopyFcn=Stateflow.SLINSF.SimulinkMan.removeBlockPreDeleteFcn  PreDeleteFcn=Stateflow.SLINSF.SimulinkMan.unsafePredeleteFcn
  Bus Creator : BusCreator  Inputs=3  OutDataTypeStr=Bus: innerLoopCmdsBus  NonVirtualBus=on
      settings: InheritFromInputs=off
  Bus Selector : BusSelector  OutputSignals=position,params
  Constant : Constant  Value=10
  Constant3 : Constant  Value=0  OutDataTypeStr=uint8
  Hdg Cmd Sat : Saturate  UpperLimit=pi  LowerLimit=-pi
      settings: AttributesFormatString=[%<UpperLimit> %<LowerLimit>]
  MATLAB Function : MATLAB Function  TreatAsAtomicUnit=on
  Mux : Mux  Inputs=2
  Selector : Selector  InputPortWidth=3  IndexOptions=Index vector (dialog)  Indices=[1 2]  OutputSizes=1
  Selector1 : Selector  InputPortWidth=4  IndexOptions=Index vector (dialog)  Indices=4  OutputSizes=1
  Selector3 : Selector  InputPortWidth=4  IndexOptions=Index vector (dialog)  Indices=4  OutputSizes=1
  Waypoint Follower : uavalgslib/Waypoint Follower  UAVType=multirotor  StartFrom=first  TransitionRadiusSource=internal  TransitionRadius=1  MinLookaheadDistance=0.1  HoverAtLastWaypoint=on  YawInput=on  ShowCrossTrackErrorOutput=off  ShowStatusOutput=off  SimulateUsing=Code generation
  Yaw Cmd Sat : Saturate  UpperLimit=pi  LowerLimit=-pi
      settings: AttributesFormatString=[%<UpperLimit> %<LowerLimit>]
  InnerLoopCmds : Outport  OutDataTypeStr=Bus: innerLoopCmdsBus
  Status : Outport  Port=2
  wires:
  Bus Creator/1 -> InnerLoopCmds/1
  Bus Selector/1 -> Selector/1  "<position>"
  Yaw Cmd Sat/1 -> Bus Creator/3  "YawCmd"
  Hdg Cmd Sat/1 -> Bus Creator/2  "HeadingCmd"
  ToWP/1 -> Bus Selector/1
  Selector1/1 -> Yaw Cmd Sat/1
  Selector3/1 -> Hdg Cmd Sat/1
  Selector/1 -> Mux/1  "LAP"
  Bus Selector/2 -> MATLAB Function/3(ToWPParam), Selector1/1, Selector3/1  "<params>"
  Ground/1 -> Mux/2
  Constant3/1 -> Status/1
  Mux/1 -> MATLAB Function/2(ToWPPos)  "LAP"
  FromWP/1 -> MATLAB Function/1(FromWP)
  Pose/1 -> Waypoint Follower/1
  MATLAB Function/1(wps) -> Waypoint Follower/2
  Constant/1 -> Waypoint Follower/3
  Waypoint Follower/1 -> Bus Creator/1  "LAP"

== system UAM_Flight_control/Flightmode/Auto/Guidance Mode Selector/GuidanceLogic.Land.Descend ==
  ToWP : Inport  OutDataTypeStr=Bus: UAVPathManagerBus
  Ground : Inport  Port=2
  Pose : Inport  Port=3
  FromWP : Inport  Port=4  OutDataTypeStr=Bus: UAVPathManagerBus
  Action Port : ActionPort
      settings: CopyFcn=Stateflow.SLINSF.SimulinkMan.removeBlockPreDeleteFcn  PreDeleteFcn=Stateflow.SLINSF.SimulinkMan.unsafePredeleteFcn
  Bus Creator : BusCreator  Inputs=3  OutDataTypeStr=Bus: innerLoopCmdsBus  NonVirtualBus=on
      settings: InheritFromInputs=off
  Bus Selector : BusSelector  OutputSignals=position,params
  Constant1 : Constant  Value=0
  Constant3 : Constant  Value=0  OutDataTypeStr=uint8
  Display3 : Display
  Hdg Cmd Sat : Saturate  UpperLimit=pi  LowerLimit=-pi
      settings: AttributesFormatString=[%<UpperLimit> %<LowerLimit>]
  MATLAB Function : MATLAB Function  TreatAsAtomicUnit=on
  MATLAB Function1 : MATLAB Function  TreatAsAtomicUnit=on
  MATLAB Function2 : MATLAB Function  TreatAsAtomicUnit=on
  MATLAB Function3 : MATLAB Function  TreatAsAtomicUnit=on
  Mux : Mux  Inputs=2
  Selector : Selector  InputPortWidth=3  IndexOptions=Index vector (dialog)  Indices=[1 2]  OutputSizes=1
  Selector1 : Selector  InputPortWidth=4  IndexOptions=Index vector (dialog)  Indices=4  OutputSizes=1
  Selector2 : Selector  InputPortWidth=4  IndexOptions=Index vector (dialog)  Indices=3  OutputSizes=1
  Selector3 : Selector  InputPortWidth=4  IndexOptions=Index vector (dialog)  Indices=4  OutputSizes=1
  Unary Minus : UnaryMinus
  Waypoint Follower : uavalgslib/Waypoint Follower  UAVType=multirotor  StartFrom=first  TransitionRadiusSource=internal  TransitionRadius=1  MinLookaheadDistance=0.1  HoverAtLastWaypoint=on  YawInput=on  ShowCrossTrackErrorOutput=off  ShowStatusOutput=off  SimulateUsing=Code generation
  Yaw Cmd Sat : Saturate  UpperLimit=pi  LowerLimit=-pi
      settings: AttributesFormatString=[%<UpperLimit> %<LowerLimit>]
  InnerLoopCmds : Outport  OutDataTypeStr=Bus: innerLoopCmdsBus
  Status : Outport  Port=2
  wires:
  Bus Creator/1 -> InnerLoopCmds/1
  Bus Selector/1 -> Selector/1  "<position>"
  Yaw Cmd Sat/1 -> Bus Creator/3  "YawCmd"
  Hdg Cmd Sat/1 -> Bus Creator/2  "HeadingCmd"
  ToWP/1 -> Bus Selector/1
  Selector1/1 -> Yaw Cmd Sat/1
  Selector3/1 -> Hdg Cmd Sat/1
  Selector/1 -> Mux/1  "LAP"
  Bus Selector/2 -> Selector1/1, Selector3/1, MATLAB Function/3(ToWPParam)  "<params>"
  Ground/1 -> Unary Minus/1, Mux/2
  Constant3/1 -> Status/1
  FromWP/1 -> MATLAB Function/1(FromWP)
  Pose/1 -> Selector2/1, MATLAB Function2/1(current_pos), Waypoint Follower/1
  MATLAB Function/1(wps) -> Waypoint Follower/2
  MATLAB Function2/1(LAP) -> Bus Creator/1
  Unary Minus/1 -> Display3/1
  Constant1/1 -> MATLAB Function1/2(land_alt)
  Selector2/1 -> MATLAB Function1/1(current_alt)  "LAP"
  MATLAB Function1/1(descent_speed) -> MATLAB Function2/2(descent_speed)

== system UAM_Flight_control/Flightmode/Auto/Guidance Mode Selector/GuidanceLogic.Land.ToLand ==
  Pose : Inport
  ToWP : Inport  Port=2  OutDataTypeStr=Bus: UAVPathManagerBus
  FromWP : Inport  Port=3  OutDataTypeStr=Bus: UAVPathManagerBus
  Action Port : ActionPort
      settings: CopyFcn=Stateflow.SLINSF.SimulinkMan.removeBlockPreDeleteFcn  PreDeleteFcn=Stateflow.SLINSF.SimulinkMan.unsafePredeleteFcn
  Bus Creator1 : BusCreator  Inputs=3  OutDataTypeStr=Bus: innerLoopCmdsBus  NonVirtualBus=on
  Constant : Constant  Value=0  OutDataTypeStr=uint8
  Lookahead Distance : Constant  OutDataTypeStr=double
  MATLAB Function : MATLAB Function  TreatAsAtomicUnit=on
  Scope : Scope
  Waypoint Follower : uavalgslib/Waypoint Follower  UAVType=multirotor  StartFrom=first  TransitionRadiusSource=internal  TransitionRadius=1  MinLookaheadDistance=0.1  HoverAtLastWaypoint=on  YawInput=on  ShowCrossTrackErrorOutput=off  ShowStatusOutput=off  SimulateUsing=Code generation
  Status : Outport
  InnerLoopCmds : Outport  Port=2  OutDataTypeStr=Bus: innerLoopCmdsBus
  wires:
  Constant/1 -> Status/1
  MATLAB Function/1(wps) -> Waypoint Follower/2
  Lookahead Distance/1 -> Waypoint Follower/3
  Bus Creator1/1 -> InnerLoopCmds/1
  ToWP/1 -> MATLAB Function/2(ToWP)
  Waypoint Follower/2 -> Bus Creator1/2  "HeadingCmd"
  FromWP/1 -> MATLAB Function/1(FromWP)
  Waypoint Follower/4 -> Scope/1
  Pose/1 -> Waypoint Follower/1
  Waypoint Follower/3 -> Bus Creator1/3  "YawCmd"
  Waypoint Follower/1 -> Bus Creator1/1  "LAP"

== system UAM_Flight_control/Flightmode/Auto/Guidance Mode Selector/GuidanceLogic.Orbit ==
  ToWP : Inport  OutDataTypeStr=Bus: UAVPathManagerBus
  Pose : Inport  Port=2
  Action Port : ActionPort
      settings: CopyFcn=Stateflow.SLINSF.SimulinkMan.removeBlockPreDeleteFcn  PreDeleteFcn=Stateflow.SLINSF.SimulinkMan.unsafePredeleteFcn
  Abs : Abs  SaturateOnIntegerOverflow=off
  Bus Creator : BusCreator  Inputs=3  OutDataTypeStr=Bus: innerLoopCmdsBus  NonVirtualBus=on
  Bus Selector : BusSelector  OutputSignals=position,params
  Data Type Conversion : DataTypeConversion  OutDataTypeStr=uint8  SaturateOnIntegerOverflow=off  RndMeth=Floor
  Lookahead Distance : Constant  Value=5  OutDataTypeStr=double
  Radius : Selector  InputPortWidth=4  IndexOptions=Index vector (dialog)  Indices=[3]  OutputSizes=1
  Relational Operator : RelationalOperator  Operator=>  OutDataTypeStr=boolean  RndMeth=Simplest  InputSameDT=off
  Sign : Signum  ZeroCross=off
  Terminator : Terminator
  Terminator1 : Terminator
  Turns : Selector  InputPortWidth=4  IndexOptions=Index vector (dialog)  Indices=[1]  OutputSizes=1
  UAV Orbit Follower : uavalgslib/Orbit Follower  UAVType=multirotor  MinOrbitRadius=1  MinLookaheadDistance=0.1  ExternalReset=none  ShowCrossTrackErrorOutput=off  ShowNumTurnsOutput=on  SimulateUsing=Code generation
  InnerLoopCmds : Outport  OutDataTypeStr=Bus: innerLoopCmdsBus
  Status : Outport  Port=2
  wires:
  Pose/1 -> UAV Orbit Follower/1
  Lookahead Distance/1 -> UAV Orbit Follower/5
  Abs/1 -> UAV Orbit Follower/3
  Bus Selector/1 -> UAV Orbit Follower/2  "<position>"
  ToWP/1 -> Bus Selector/1
  Bus Creator/1 -> InnerLoopCmds/1
  UAV Orbit Follower/2 -> Bus Creator/2  "HeadingCmd"
  UAV Orbit Follower/3 -> Bus Creator/3  "YawCmd"
  Bus Selector/2 -> Turns/1, Radius/1  "<params>"
  Radius/1 -> Abs/1, Sign/1
  Sign/1 -> UAV Orbit Follower/4
  Relational Operator/1 -> Data Type Conversion/1
  Turns/1 -> Relational Operator/2
  Data Type Conversion/1 -> Status/1
  UAV Orbit Follower/6 -> Relational Operator/1
  UAV Orbit Follower/4 -> Terminator/1
  UAV Orbit Follower/5 -> Terminator1/1
  UAV Orbit Follower/1 -> Bus Creator/1  "LAP"

== system UAM_Flight_control/Flightmode/Auto/Guidance Mode Selector/GuidanceLogic.Takeoff ==
  ToWP : Inport  OutDataTypeStr=Bus: UAVPathManagerBus
  Pose : Inport  Port=2
  Action Port : ActionPort
      settings: CopyFcn=Stateflow.SLINSF.SimulinkMan.removeBlockPreDeleteFcn  PreDeleteFcn=Stateflow.SLINSF.SimulinkMan.unsafePredeleteFcn
  Bus Creator : BusCreator  Inputs=3  OutDataTypeStr=Bus: innerLoopCmdsBus  NonVirtualBus=on
      settings: InheritFromInputs=off
  Bus Selector : BusSelector  OutputSignals=position,params
  Constant : Constant  Value=0  OutDataTypeStr=uint8
  Constant2 : Constant
  Demux : Demux  Outputs=[2 1 1]
  Demux1 : Demux  Outputs=[2 1]
  Hdg. Cmd Sat : Saturate  UpperLimit=pi  LowerLimit=-pi
      settings: AttributesFormatString=[%<UpperLimit> %<LowerLimit>]
  Mux : Mux  Inputs=2
  Selector3 : Selector  InputPortWidth=4  IndexOptions=Index vector (dialog)  Indices=1  OutputSizes=1
  Switch : Switch  Criteria=u2 > Threshold  SaturateOnIntegerOverflow=off  InputSameDT=off
  Terminator : Terminator
  Terminator1 : Terminator
  Unit Delay : UnitDelay  SampleTime=-1  HasFrameUpgradeWarning=on
  Unit Delay1 : UnitDelay  SampleTime=-1  HasFrameUpgradeWarning=on
  Yaw Cmd Sat : Saturate  UpperLimit=pi  LowerLimit=-pi
      settings: AttributesFormatString=[%<UpperLimit> %<LowerLimit>]
  InnerLoopCmds : Outport  OutDataTypeStr=Bus: innerLoopCmdsBus
  Status : Outport  Port=2
  wires:
  Hdg. Cmd Sat/1 -> Bus Creator/2  "HeadingCmd"
  Bus Creator/1 -> InnerLoopCmds/1
  Constant/1 -> Status/1
  Pose/1 -> Demux/1
  Yaw Cmd Sat/1 -> Bus Creator/3  "YawCmd"
  ToWP/1 -> Bus Selector/1
  Bus Selector/2 -> Selector3/1  "<params>"
  Bus Selector/1 -> Demux1/1  "<position>"
  Selector3/1 -> Hdg. Cmd Sat/1
  Unit Delay/1 -> Switch/2
  Constant2/1 -> Unit Delay/1
  Unit Delay1/1 -> Switch/1
  Switch/1 -> Unit Delay1/1, Yaw Cmd Sat/1
  Demux/3 -> Switch/3
  Demux1/2 -> Mux/2
  Demux1/1 -> Terminator/1
  Demux/2 -> Terminator1/1
  Mux/1 -> Bus Creator/1  "LAP"
  Demux/1 -> Mux/1

== system UAM_Flight_control/Flightmode/Auto/Guidance Mode Selector/GuidanceLogic.WP ==
  FromWP : Inport  OutDataTypeStr=Bus: UAVPathManagerBus
  Pose : Inport  Port=2
  ToWP : Inport  Port=3  OutDataTypeStr=Bus: UAVPathManagerBus
  Action Port : ActionPort
      settings: CopyFcn=Stateflow.SLINSF.SimulinkMan.removeBlockPreDeleteFcn  PreDeleteFcn=Stateflow.SLINSF.SimulinkMan.unsafePredeleteFcn
  Back Transition Guard : Subsystem
  Bus Creator : BusCreator  Inputs=3  OutDataTypeStr=Bus: innerLoopCmdsBus  NonVirtualBus=on
  Bus Creator1 : BusCreator  Inputs=1
  Bus Creator2 : BusCreator  Inputs=3
  Bus Selector : BusSelector  OutputSignals=position
  Constant1 : Constant  Value=2
  Data Type Conversion : DataTypeConversion  OutDataTypeStr=uint8  SaturateOnIntegerOverflow=off  RndMeth=Floor
  Data Type Conversion1 : DataTypeConversion  OutDataTypeStr=double  SaturateOnIntegerOverflow=off  RndMeth=Floor
  Data Type Conversion2 : DataTypeConversion  OutDataTypeStr=double  SaturateOnIntegerOverflow=off  RndMeth=Floor
  Demux : Demux  Outputs=3
  Dist2WP : Subsystem
  Lookahead Distance : Constant  OutDataTypeStr=double
  MATLAB Function : MATLAB Function  TreatAsAtomicUnit=on
  Relational Operator : RelationalOperator  OutDataTypeStr=boolean  RndMeth=Simplest  InputSameDT=off
  Scope : Scope
  Selector : Selector  InputPortWidth=3  IndexOptions=Index vector (dialog)  Indices=3  OutputSizes=1
  Terminator : Terminator
  Waypoint Follower : uavalgslib/Waypoint Follower  UAVType=multirotor  StartFrom=closest  TransitionRadiusSource=internal  TransitionRadius=R_WAYPOINTTRANSITION*3  MinLookaheadDistance=0.1  HoverAtLastWaypoint=off  YawInput=on  ShowCrossTrackErrorOutput=off  ShowStatusOutput=off  SimulateUsing=Code generation
  Yaw Cmd Sat : Saturate  UpperLimit=pi  LowerLimit=-pi
      settings: AttributesFormatString=[%<UpperLimit> %<LowerLimit>]
  InnerLoopCmds : Outport  OutDataTypeStr=Bus: innerLoopCmdsBus
  Status : Outport  Port=2
  wires:
  Data Type Conversion/1 -> Status/1
  Bus Creator/1 -> InnerLoopCmds/1
  ToWP/1 -> Dist2WP/3(ToWP), Bus Selector/1, MATLAB Function/2(ToWP)
  MATLAB Function/1(wps) -> Waypoint Follower/2
  Waypoint Follower/2 -> Bus Creator/2  "HeadingCmd"
  Waypoint Follower/4 -> Scope/1
  Dist2WP/1(Dist) -> Relational Operator/2
  FromWP/1 -> Back Transition Guard/2(FromWP)
  Relational Operator/1 -> Data Type Conversion/1
  Back Transition Guard/1(PrevWP) -> Dist2WP/2(FromWP), MATLAB Function/1(FromWP)
  Pose/1 -> Back Transition Guard/1(Poses), Waypoint Follower/1, Dist2WP/1(Pose)
  Lookahead Distance/1 -> Waypoint Follower/3
  Waypoint Follower/3 -> Yaw Cmd Sat/1  "YawCmd"
  Yaw Cmd Sat/1 -> Bus Creator/3  "YawCmd"
  Constant1/1 -> Relational Operator/1
  Bus Creator1/1 -> Data Type Conversion1/1  "LAP"
  Waypoint Follower/1 -> Demux/1  "LAP"
  Data Type Conversion1/1 -> Selector/1  "LAP"
  Demux/1 -> Bus Creator2/1  "X"
  Demux/2 -> Bus Creator2/2  "Y"
  Bus Creator2/1 -> Data Type Conversion2/1  "LAP"
  Data Type Conversion2/1 -> Bus Creator/1  "LAP"
  Bus Selector/1 -> Bus Creator1/1  "<position>"
  Selector/1 -> Bus Creator2/3  "Z"
  Demux/3 -> Terminator/1
